simulink model "ysw_PID1"  (R2014a)
settings: Solver=ode45  StartTime=0.0  StopTime=10  RelTol=1e-3
undefined symbols (not defined in the file or in its folder): den, num
settings Model: Creator=ii  LastModifiedBy=ii
settings SolverCC: ZeroCrossAlgorithm=Adaptive
settings DebuggingCC: UnderspecifiedInitializationDetection=Classic

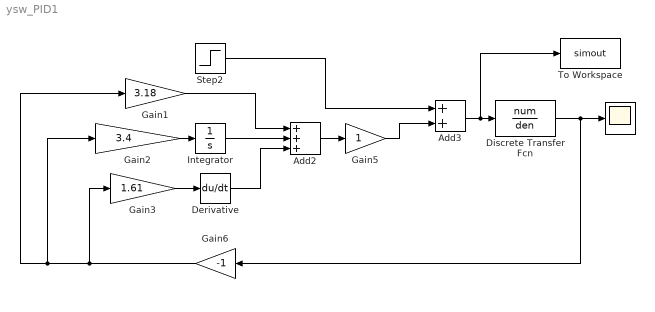
== system ysw_PID1 ==
  " " : Scope
  Add2 : Sum  Inputs=+++
  Add3 : Sum
  Derivative : Derivative
  Discrete Transfer Fcn : DiscreteTransferFcn  Numerator=num  Denominator=den  SampleTime=0.001
  Gain1 : Gain  Gain=3.18
  Gain2 : Gain  Gain=3.4
  Gain3 : Gain  Gain=1.61
  Gain5 : Gain
  Gain6 : Gain  Gain=-1
  Integrator : Integrator
  Step2 : Step  Time=0  SampleTime=0.001
  To Workspace : ToWorkspace  VariableName=simout  SampleTime=0.001
  wires:
  Step2/1 -> Add3/1
  Gain1/1 -> Add2/1
  Gain2/1 -> Integrator/1
  Integrator/1 -> Add2/2
  Gain3/1 -> Derivative/1
  Derivative/1 -> Add2/3
  Add2/1 -> Gain5/1
  Gain5/1 -> Add3/2
  Discrete Transfer Fcn/1 -> Gain6/1, " "/1
  Gain6/1 -> Gain3/1, Gain2/1, Gain1/1
  Add3/1 -> To Workspace/1, Discrete Transfer Fcn/1
